simulink model "SS_Error_space"  (R2021a)
settings: Solver=ode45  StartTime=0.0  StopTime=10  FixedStep=0.0001  RelTol=1e-3
undefined symbols (not defined in the file): degs2rpm, drv, err_space, est_par, gbox, mot, rads2rpm, rpm2rads, sens
settings Model: Creator=gioel  LastModifiedBy=gioel
settings DataIOCC: ReturnWorkspaceOutputs=off

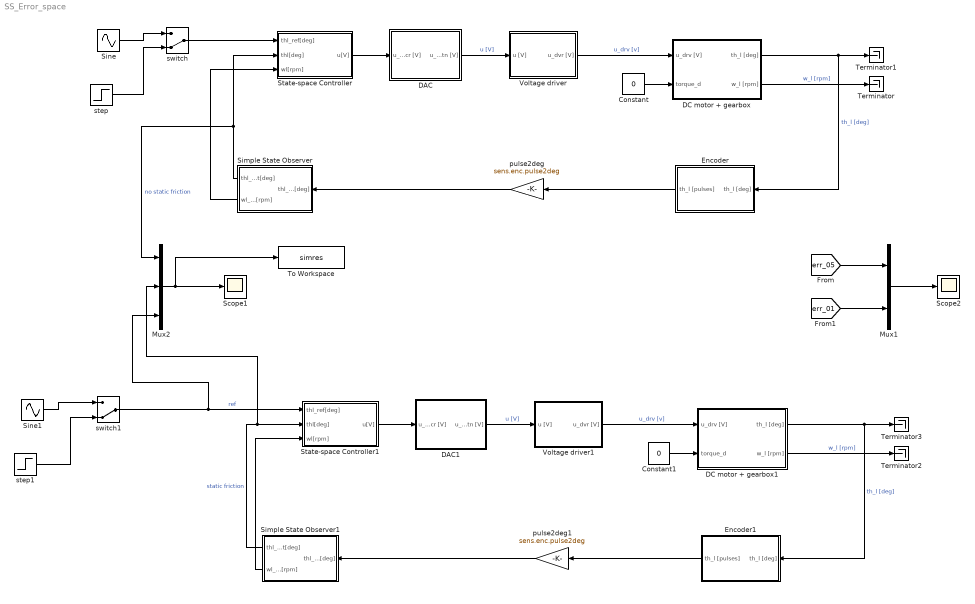
== system SS_Error_space ==
  Constant : Constant  Value=0
  Constant1 : Constant  Value=0
  DAC : Subsystem
  DAC1 : Subsystem
  DC motor + gearbox : Subsystem
  DC motor + gearbox1 : Subsystem
  Encoder : Subsystem
  Encoder1 : Subsystem
  Mux1 : Mux  Inputs=2
  Mux2 : Mux  Inputs=3
  Scope1 : Scope
  Scope2 : Scope
  Simple State Observer : Subsystem
  Simple State Observer1 : Subsystem
  Sine : Sin  Amplitude=40  Frequency=2*pi/0.1  SampleTime=0
  Sine1 : Sin  Amplitude=40  Frequency=2*pi/0.1  SampleTime=0
  State-space Controller : Subsystem
  State-space Controller1 : Subsystem
  Terminator{,1..3} (4 alike) : Terminator
  To Workspace : ToWorkspace  VariableName=simres  SaveFormat=Structure With Time  SampleTime=-1
  Voltage driver : Subsystem
  Voltage driver1 : Subsystem
  pulse2deg : Gain  Gain=sens.enc.pulse2deg
  pulse2deg1 : Gain  Gain=sens.enc.pulse2deg
  step : Step  Time=0  After=40  SampleTime=0
  step1 : Step  Time=0  After=40  SampleTime=0
  switch : ManualSwitch  CurrentSetting=0
  switch1 : ManualSwitch  CurrentSetting=0
  wires:
  Simple State Observer/2(wl_est[rpm]) -> State-space Controller/3(wl[rpm])
  DAC1/1(u_cntn [V]) -> Voltage driver1/1(u [V])  "u [V]"
  Constant1/1 -> DC motor + gearbox1/2(torque_d)
  pulse2deg/1 -> Simple State Observer/1(thl_meas[deg])
  Simple State Observer/1(thl_est[deg]) -> State-space Controller/2(thl[deg]), Mux2/1  "no static friction"
  Voltage driver1/1(u_dvr [V]) -> DC motor + gearbox1/1(u_drv [V])  "u_drv [v]"
  DC motor + gearbox/2(w_l [rpm]) -> Terminator/1  "w_l [rpm]"
  Constant/1 -> DC motor + gearbox/2(torque_d)
  DAC/1(u_cntn [V]) -> Voltage driver/1(u [V])  "u [V]"
  Encoder1/1(th_l [pulses]) -> pulse2deg1/1
  pulse2deg1/1 -> Simple State Observer1/1(thl_meas[deg])
  DC motor + gearbox1/1(th_l [deg]) -> Terminator3/1, Encoder1/1(th_l [deg])  "th_l [deg]"
  switch1/1 -> State-space Controller1/1(thl_ref[deg]), Mux2/3  "ref"
  Voltage driver/1(u_dvr [V]) -> DC motor + gearbox/1(u_drv [V])  "u_drv [v]"
  DC motor + gearbox/1(th_l [deg]) -> Terminator1/1, Encoder/1(th_l [deg])  "th_l [deg]"
  Mux2/1 -> To Workspace/1, Scope1/1
  State-space Controller/1(u[V]) -> DAC/1(u_dscr [V])
  DC motor + gearbox1/2(w_l [rpm]) -> Terminator2/1  "w_l [rpm]"
  Encoder/1(th_l [pulses]) -> pulse2deg/1
  Simple State Observer1/1(thl_est[deg]) -> Mux2/2, State-space Controller1/2(thl[deg])  "static friction"
  State-space Controller1/1(u[V]) -> DAC1/1(u_dscr [V])
  Simple State Observer1/2(wl_est[rpm]) -> State-space Controller1/3(wl[rpm])
  [err_05] -> Mux1/1
  [err_01] -> Mux1/2
  Mux1/1 -> Scope2/1
  Sine/1 -> switch/1
  switch/1 -> State-space Controller/1(thl_ref[deg])
  step/1 -> switch/2
  Sine1/1 -> switch1/1
  step1/1 -> switch1/2

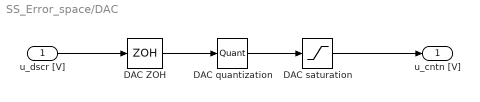
== system SS_Error_space/DAC ==
  u_dscr [V] : Inport
  DAC ZOH : ZeroOrderHold  SampleTime=sens.enc.T_s
  DAC quantization : Quantizer  QuantizationInterval=daq.dac.q
  DAC saturation : Saturate  UpperLimit=10  LowerLimit=-10
  u_cntn [V] : Outport
  wires:
  DAC quantization/1 -> DAC saturation/1
  DAC ZOH/1 -> DAC quantization/1
  DAC saturation/1 -> u_cntn [V]/1
  u_dscr [V]/1 -> DAC ZOH/1

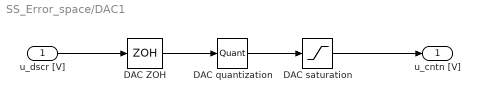
== system SS_Error_space/DAC1 ==
  u_dscr [V] : Inport
  DAC ZOH : ZeroOrderHold  SampleTime=sens.enc.T_s
  DAC quantization : Quantizer  QuantizationInterval=daq.dac.q
  DAC saturation : Saturate  UpperLimit=10  LowerLimit=-10
  u_cntn [V] : Outport
  wires:
  DAC quantization/1 -> DAC saturation/1
  DAC ZOH/1 -> DAC quantization/1
  DAC saturation/1 -> u_cntn [V]/1
  u_dscr [V]/1 -> DAC ZOH/1

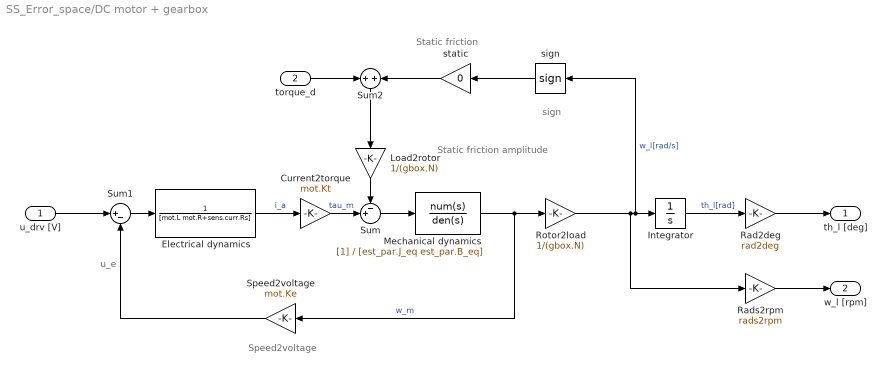
== system SS_Error_space/DC motor + gearbox ==
  note: u_e
  note: Speed2voltage
  note: Static friction
  note: sign
  note: Static friction
      |  amplitude
  u_drv [V] : Inport
  torque_d : Inport  Port=2
  Current2torque : Gain  Gain=mot.Kt
  Electrical dynamics : TransferFcn  Denominator=[mot.L mot.R+sens.curr.Rs]
  Integrator : Integrator
  Load2rotor : Gain  Gain=1/(gbox.N)
  Mechanical dynamics : TransferFcn  Denominator=[est_par.J_eq est_par.B_eq]
  Rad2deg : Gain  Gain=rad2deg
  Rads2rpm : Gain  Gain=rads2rpm
  Rotor2load : Gain  Gain=1/(gbox.N)
  Speed2voltage : Gain  Gain=mot.Ke
  Sum : Sum  Inputs=-+|
  Sum1 : Sum  Inputs=|+-
  Sum2 : Sum  Inputs=+|+
  sign : Signum  ZeroCross=off
  static : Gain  Gain=0
  th_l [deg] : Outport
  w_l [rpm] : Outport  Port=2
  wires:
  u_drv [V]/1 -> Sum1/1
  Rads2rpm/1 -> w_l [rpm]/1
  Electrical dynamics/1 -> Current2torque/1  "i_a"
  Current2torque/1 -> Sum/2  "tau_m"
  Rad2deg/1 -> th_l [deg]/1
  sign/1 -> static/1
  Sum1/1 -> Electrical dynamics/1
  Integrator/1 -> Rad2deg/1  "th_l[rad]"
  Sum/1 -> Mechanical dynamics/1
  Load2rotor/1 -> Sum/1
  Speed2voltage/1 -> Sum1/2
  Rotor2load/1 -> sign/1, Integrator/1, Rads2rpm/1  "w_l[rad/s]"
  Mechanical dynamics/1 -> Speed2voltage/1, Rotor2load/1  "w_m"
  Sum2/1 -> Load2rotor/1
  torque_d/1 -> Sum2/1
  static/1 -> Sum2/2

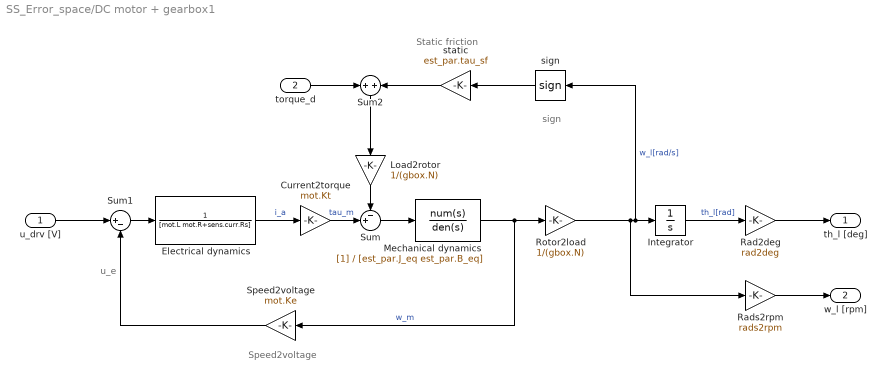
== system SS_Error_space/DC motor + gearbox1 ==
  note: u_e
  note: Speed2voltage
  note: Static friction
  note: sign
  u_drv [V] : Inport
  torque_d : Inport  Port=2
  Current2torque : Gain  Gain=mot.Kt
  Electrical dynamics : TransferFcn  Denominator=[mot.L mot.R+sens.curr.Rs]
  Integrator : Integrator
  Load2rotor : Gain  Gain=1/(gbox.N)
  Mechanical dynamics : TransferFcn  Denominator=[est_par.J_eq est_par.B_eq]
  Rad2deg : Gain  Gain=rad2deg
  Rads2rpm : Gain  Gain=rads2rpm
  Rotor2load : Gain  Gain=1/(gbox.N)
  Speed2voltage : Gain  Gain=mot.Ke
  Sum : Sum  Inputs=-+|
  Sum1 : Sum  Inputs=|+-
  Sum2 : Sum  Inputs=+|+
  sign : Signum  ZeroCross=off
  static : Gain  Gain=est_par.tau_sf
  th_l [deg] : Outport
  w_l [rpm] : Outport  Port=2
  wires:
  u_drv [V]/1 -> Sum1/1
  Rads2rpm/1 -> w_l [rpm]/1
  Electrical dynamics/1 -> Current2torque/1  "i_a"
  Current2torque/1 -> Sum/2  "tau_m"
  Rad2deg/1 -> th_l [deg]/1
  sign/1 -> static/1
  Sum1/1 -> Electrical dynamics/1
  Integrator/1 -> Rad2deg/1  "th_l[rad]"
  Sum/1 -> Mechanical dynamics/1
  Load2rotor/1 -> Sum/1
  Speed2voltage/1 -> Sum1/2
  Rotor2load/1 -> sign/1, Integrator/1, Rads2rpm/1  "w_l[rad/s]"
  Mechanical dynamics/1 -> Speed2voltage/1, Rotor2load/1  "w_m"
  Sum2/1 -> Load2rotor/1
  torque_d/1 -> Sum2/1
  static/1 -> Sum2/2

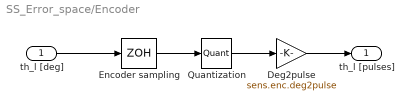
== system SS_Error_space/Encoder ==
  th_l [deg] : Inport
  Deg2pulse : Gain  Gain=sens.enc.deg2pulse
  Encoder sampling : ZeroOrderHold  SampleTime=0.001
  Quantization : Quantizer  QuantizationInterval=sens.enc.q
  th_l [pulses] : Outport
  wires:
  Encoder sampling/1 -> Quantization/1
  Quantization/1 -> Deg2pulse/1
  th_l [deg]/1 -> Encoder sampling/1
  Deg2pulse/1 -> th_l [pulses]/1

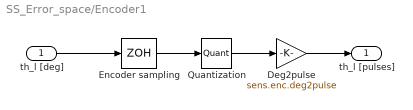
== system SS_Error_space/Encoder1 ==
  th_l [deg] : Inport
  Deg2pulse : Gain  Gain=sens.enc.deg2pulse
  Encoder sampling : ZeroOrderHold  SampleTime=0.001
  Quantization : Quantizer  QuantizationInterval=sens.enc.q
  th_l [pulses] : Outport
  wires:
  Encoder sampling/1 -> Quantization/1
  Quantization/1 -> Deg2pulse/1
  th_l [deg]/1 -> Encoder sampling/1
  Deg2pulse/1 -> th_l [pulses]/1

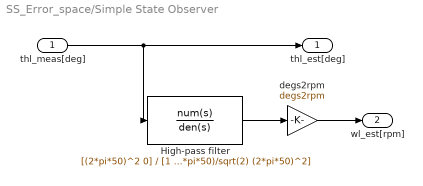
== system SS_Error_space/Simple State Observer ==
  thl_meas[deg] : Inport
  High-pass filter : TransferFcn  Numerator=[(2*pi*50)^2 0]  Denominator=[1 (2*2*pi*50)/sqrt(2) (2*pi*50)^2]
  degs2rpm : Gain  Gain=degs2rpm
  thl_est[deg] : Outport
  wl_est[rpm] : Outport  Port=2
  wires:
  High-pass filter/1 -> degs2rpm/1
  degs2rpm/1 -> wl_est[rpm]/1
  thl_meas[deg]/1 -> thl_est[deg]/1, High-pass filter/1

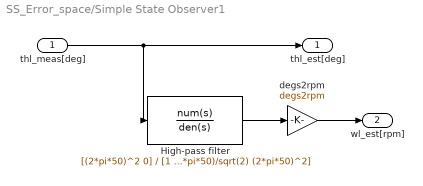
== system SS_Error_space/Simple State Observer1 ==
  thl_meas[deg] : Inport
  High-pass filter : TransferFcn  Numerator=[(2*pi*50)^2 0]  Denominator=[1 (2*2*pi*50)/sqrt(2) (2*pi*50)^2]
  degs2rpm : Gain  Gain=degs2rpm
  thl_est[deg] : Outport
  wl_est[rpm] : Outport  Port=2
  wires:
  High-pass filter/1 -> degs2rpm/1
  degs2rpm/1 -> wl_est[rpm]/1
  thl_meas[deg]/1 -> thl_est[deg]/1, High-pass filter/1

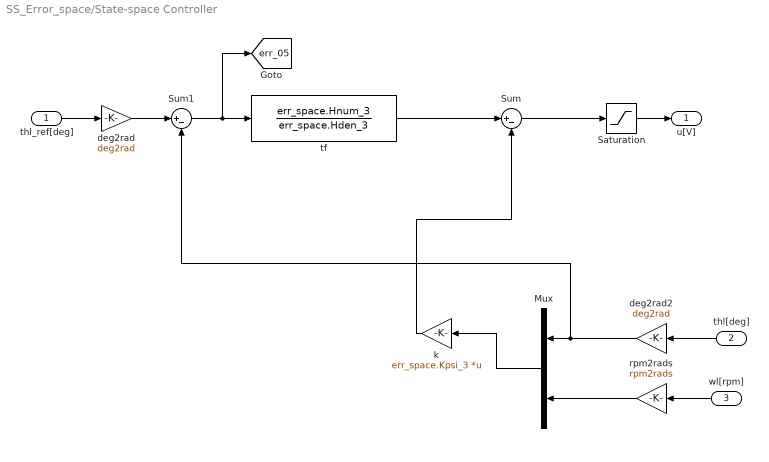
== system SS_Error_space/State-space Controller ==
  thl_ref[deg] : Inport
  thl[deg] : Inport  Port=2
  wl[rpm] : Inport  Port=3
  Mux : Mux  Inputs=2
  Saturation : Saturate  UpperLimit=10  LowerLimit=-10
  Sum : Sum  Inputs=|+-
  Sum1 : Sum  Inputs=|+-
  deg2rad : Gain  Gain=deg2rad
  deg2rad2 : Gain  Gain=deg2rad
  k : Gain  Gain=err_space.Kpsi_3  Multiplication=Matrix(K*u)
  rpm2rads : Gain  Gain=rpm2rads
  tf : TransferFcn  Numerator=err_space.Hnum_3  Denominator=err_space.Hden_3
  u[V] : Outport
  tag scope: err_05=global
  wires:
  thl_ref[deg]/1 -> deg2rad/1
  wl[rpm]/1 -> rpm2rads/1
  thl[deg]/1 -> deg2rad2/1
  Saturation/1 -> u[V]/1
  Sum/1 -> Saturation/1
  tf/1 -> Sum/1
  deg2rad2/1 -> Sum1/2, Mux/1
  rpm2rads/1 -> Mux/2
  Mux/1 -> k/1
  k/1 -> Sum/2
  deg2rad/1 -> Sum1/1
  Sum1/1 -> [err_05], tf/1

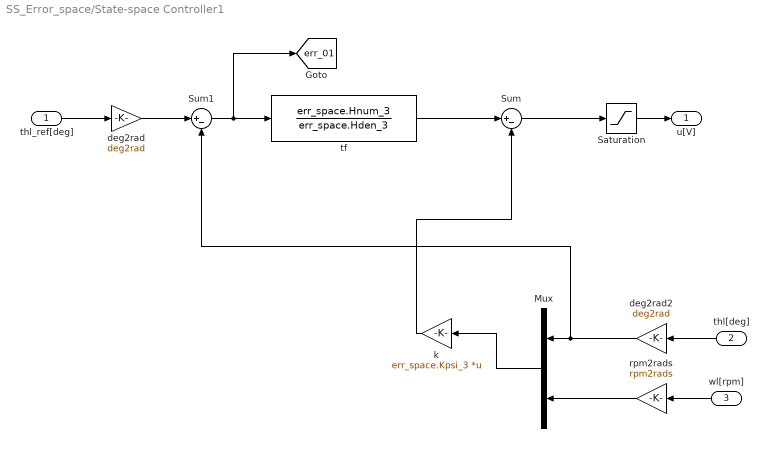
== system SS_Error_space/State-space Controller1 ==
  thl_ref[deg] : Inport
  thl[deg] : Inport  Port=2
  wl[rpm] : Inport  Port=3
  Mux : Mux  Inputs=2
  Saturation : Saturate  UpperLimit=10  LowerLimit=-10
  Sum : Sum  Inputs=|+-
  Sum1 : Sum  Inputs=|+-
  deg2rad : Gain  Gain=deg2rad
  deg2rad2 : Gain  Gain=deg2rad
  k : Gain  Gain=err_space.Kpsi_3  Multiplication=Matrix(K*u)
  rpm2rads : Gain  Gain=rpm2rads
  tf : TransferFcn  Numerator=err_space.Hnum_3  Denominator=err_space.Hden_3
  u[V] : Outport
  tag scope: err_01=global
  wires:
  deg2rad2/1 -> Sum1/2, Mux/1
  Mux/1 -> k/1
  tf/1 -> Sum/1
  thl_ref[deg]/1 -> deg2rad/1
  wl[rpm]/1 -> rpm2rads/1
  thl[deg]/1 -> deg2rad2/1
  Saturation/1 -> u[V]/1
  Sum/1 -> Saturation/1
  rpm2rads/1 -> Mux/2
  k/1 -> Sum/2
  deg2rad/1 -> Sum1/1
  Sum1/1 -> [err_01], tf/1

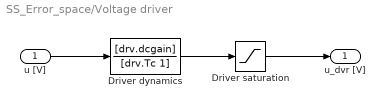
== system SS_Error_space/Voltage driver ==
  u [V] : Inport
  Driver dynamics : TransferFcn  Numerator=[drv.dcgain]  Denominator=[drv.Tc 1]
  Driver saturation : Saturate  UpperLimit=12  LowerLimit=-12
  u_dvr [V] : Outport
  wires:
  Driver saturation/1 -> u_dvr [V]/1
  Driver dynamics/1 -> Driver saturation/1
  u [V]/1 -> Driver dynamics/1

== system SS_Error_space/Voltage driver1 ==
  u [V] : Inport
  Driver dynamics : TransferFcn  Numerator=[drv.dcgain]  Denominator=[drv.Tc 1]
  Driver saturation : Saturate  UpperLimit=12  LowerLimit=-12
  u_dvr [V] : Outport
  wires:
  Driver saturation/1 -> u_dvr [V]/1
  Driver dynamics/1 -> Driver saturation/1
  u [V]/1 -> Driver dynamics/1
